simulink model "InvPen_Model"  (R2024b)
settings: Solver=VariableStepAuto  StartTime=0.0  StopTime=9.0  RelTol=1e-3
values from neighbouring files (symbols this model uses):
  b = 0.1    [InvPen_Values.m]
  g = 9.8    [InvPen_Values.m]
  I = 0.006    [InvPen_Values.m]
  l = 0.3    [InvPen_Values.m]
  m = 0.2    [InvPen_Values.m]
  M = 0.5    [InvPen_Values.m]
undefined symbols (not defined in the file or in its folder): Kd, Ki, Kp
libraries: slpidlib x1
settings Model: Creator=Arghya  LastModifiedBy=Arghya

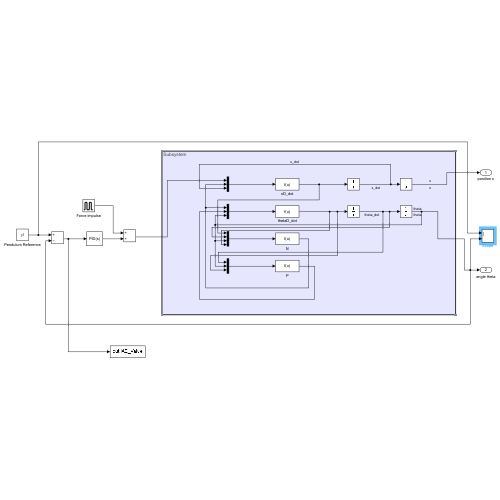
[thumbnail: Simulink's stored preview of the top-level diagram]
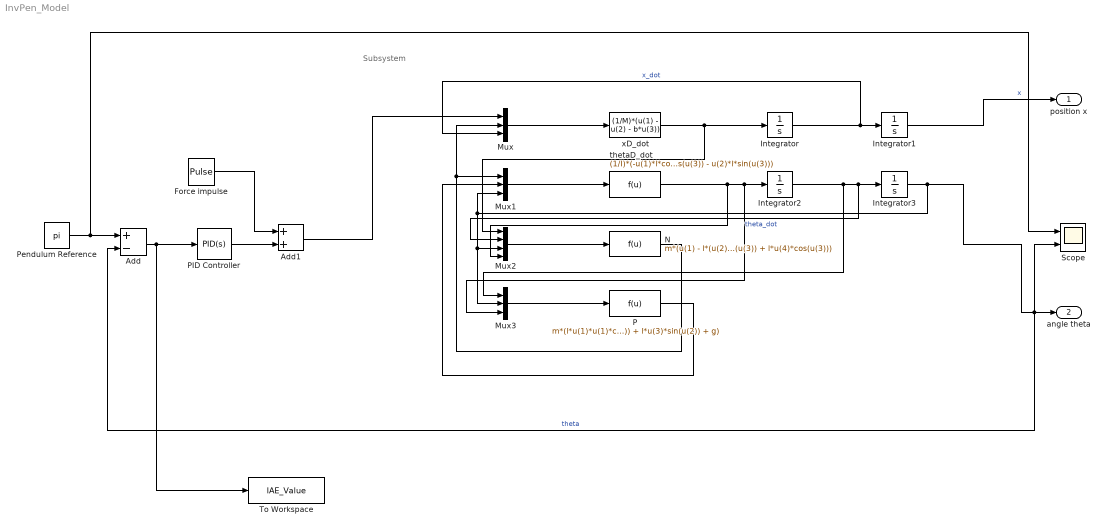
== system InvPen_Model ==
  note: Subsystem
  Add : Sum  Inputs=+-
  Add1 : Sum
  Force impulse : DiscretePulseGenerator  PulseType=Time based  Period=10  PulseWidth=5
  Integrator : Integrator  ContinuousStateAttributes="\"x_dot\""
  Integrator1 : Integrator  ContinuousStateAttributes="\"x\""
  Integrator2 : Integrator  ContinuousStateAttributes="\"theta_dot\""
  Integrator3 : Integrator  InitialCondition=pi  ContinuousStateAttributes="\"theta\""
  Mux : Mux  Inputs=3
  Mux1 : Mux  Inputs=3
  Mux2 : Mux
  Mux3 : Mux  Inputs=3
  N : Fcn  Expr=m*(u(1) - l*(u(2)^2)*sin(u(3)) + l*u(4)*cos(u(3)))
  P : Fcn  Expr=m*(l*u(1)*u(1)*cos(u(2)) + l*u(3)*sin(u(2)) + g)
  PID Controller : slpidlib/PID Controller  Controller=PID  Form=Parallel  TimeDomain=Continuous-time  UseExternalTs=off  SampleTime=-1  IntegratorMethod=Forward Euler  FilterMethod=Forward Euler  ControllerParametersSource=internal  P=Kp  I=Ki  UseKiTs=off  D=Kd  UseExternalDerivativeSource=off  N=100  UseFilter=on  TunerSelectOption=Transfer Function Based (PID Tuner App)  InitialConditionSource=internal  InitialConditionForIntegrator=0  InitialConditionForFilter=0  DifferentiatorICPrevScaledInput=0  ExternalReset=none  TrackingMode=off  Kt=1  LimitOutput=off  SatLimitsSource=internal  UpperSaturationLimit=inf  LowerSaturationLimit=-inf  LinearizeAsGain=on  AntiWindupMode=none  Kb=1  LimitIntegrator=off  UpperIntegratorSaturationLimit=inf  LowerIntegratorSaturationLimit=-inf  POutMin=[]  POutMax=[]  IOutMin=[]  IOutMax=[]  DOutMin=[]  DOutMax=[]  NOutMin=[]  NOutMax=[]  SumOutMin=[]  SumOutMax=[]  SaturationOutMin=[]  SaturationOutMax=[]  PParamMin=[]  PParamMax=[]  IParamMin=[]  IParamMax=[]  DParamMin=[]  DParamMax=[]  NParamMin=[]  NParamMax=[]  KbParamMin=[]  KbParamMax=[]  KtParamMin=[]  KtParamMax=[]  KbOutMin=[]  KbOutMax=[]  KtOutMin=[]  KtOutMax=[]  IntegratorOutMin=[]  IntegratorOutMax=[]  FilterOutMin=[]  FilterOutMax=[]  SumI1OutMin=[]  SumI1OutMax=[]  SumI2OutMin=[]  SumI2OutMax=[]  SumI3OutMin=[]  SumI3OutMax=[]  SumI4OutMin=[]  SumI4OutMax=[]  SumDOutMin=[]  SumDOutMax=[]  DifferentiatorOutMin=[]  DifferentiatorOutMax=[]  FilterDiffOutCoefMin=[]  FilterDiffOutCoefMax=[]  ReciprocalOutMin=[]  ReciprocalOutMax=[]  SumDenOutMin=[]  SumDenOutMax=[]  SumNumOutMin=[]  SumNumOutMax=[]  DivideOutMin=[]  DivideOutMax=[]  UdiffTsProdOutMin=[]  UdiffTsProdOutMax=[]  NTsProdOutMin=[]  NTsProdOutMax=[]  UintegralTsProdOutMin=[]  UintegralTsProdOutMax=[]  UngainTsProdOutMin=[]  UngainTsProdOutMax=[]  ClampingZeroOutDataTypeStr=Inherit: Inherit via back propagation  ClampingZeroOutMin=[]  ClampingZeroOutMax=[]  FilterDenConstantOutDataTypeStr=Inherit: Inherit via back propagation  FilterDenConstantOutMin=[]  FilterDenConstantOutMax=[]  PCopyOutDataTypeStr=Inherit: Inherit via back propagation  PCopyOutMin=[]  PCopyOutMax=[]  NCopyOutDataTypeStr=Inherit: Inherit via back propagation  NCopyOutMin=[]  NCopyOutMax=[]  IntegratorContinuousStateAttributes=''  IntegratorStateMustResolveToSignalObject=off  IntegratorRTWStateStorageClass=Auto  FilterContinuousStateAttributes=''  FilterStateMustResolveToSignalObject=off  FilterRTWStateStorageClass=Auto  ParallelPVariant=InternalParameters  IdealPVariant=Disabled  IVariant=InternalParameters  DVariant=InternalParameters  IntegratorVariant=Continuous  SatVariant=Disabled  AWVariant=Passthrough  PCopyVariant=Disabled  TRVariant=Disabled  FdbkBlocksVariant=Forward  IdealPFdbkVariant=Disabled  SatFdbkVariant=Disabled  DerivativeFilterVariant=ContFilter  NVariant=InternalParameters  NCopyVariant=Disabled  FilterICVariant=InternalICsFilter  IntegratorICVariant=InternalICs  ExternalResetVariant=Disabled  TRSumVariant=Passthrough  SumFdbkVariant=Disabled  SumVariant=Sum_PID  TsampFilterVariant=InternalTs  TsampNgainVariant=Passthrough  TsampIntegralVariant=Disabled_SignalSpec  ExternalSaturationOutDataTypeStr=Inherit: Same as second input  DerivativeSourceVariant=ErrorSignal  PreIntVariant=InternalPreInt
  Pendulum Reference : Constant  Value=pi  SampleTime=9.0
  Scope : Scope  NumInputPorts=2
  To Workspace : ToWorkspace  VariableName=IAE_Value  SampleTime=-1
      settings: Save2DSignal=2-D array (concatenate along first dimension)
  thetaD_dot : Fcn  Expr=(1/I)*(-u(1)*l*cos(u(3)) - u(2)*l*sin(u(3)))
  xD_dot : Fcn  Expr=(1/M)*(u(1) - u(2) - b*u(3))
  position x : Outport
  angle theta : Outport  Port=2
  wires:
  PID Controller/1 -> Add1/2
  Add/1 -> To Workspace/1, PID Controller/1
  Pendulum Reference/1 -> Scope/1, Add/1
  Force impulse/1 -> Add1/1
  Integrator1/1 -> position x/1  "x"
  Mux2/1 -> N/1
  thetaD_dot/1 -> Mux2/4, Mux3/3, Integrator2/1
  Mux1/1 -> thetaD_dot/1
  P/1 -> Mux1/2
  Mux/1 -> xD_dot/1
  N/1 -> Mux1/1, Mux/2
  Integrator/1 -> Mux/3, Integrator1/1  "x_dot"
  Integrator2/1 -> Mux3/1, Mux2/2, Integrator3/1  "theta_dot"
  Integrator3/1 -> Mux3/2, Mux2/3, Mux1/3, Scope/2, Add/2, angle theta/1  "theta"
  xD_dot/1 -> Mux2/1, Integrator/1
  Mux3/1 -> P/1
  Add1/1 -> Mux/1
